simulink model "tta_ut"  (Simulink 8.1)
settings: Solver=ode1  StartTime=0.0  StopTime=Inf  FixedStep=0.001  RelTol=1e-3
PostLoadFcn:
  | , if any(exist('dsrtsu_mdlpostloadfcn', 'file') == [2, 3, 6]), try dsrtsu_mdlpostloadfcn('Execute', bdroot); catch fprintf('Error in PostLoadFcn (dsrtsu_mdlpostloadfcn) for model "%s":\n %s\n', bdroot, lasterr); end, end,
undefined symbols (not defined in the file or in its folder): KIFO_OffsetToBumper_m
libraries: siltestlib x5, tta x1
settings Model: DSRTSU_INTERNAL_RTI_VER=450  DSRTSU_INTERNAL_RTI_TYPE=rti1401  RTICANMMDATA=struct('GeneralSetupData',struct('modelroot','D:\PROJECTS\HAITEC\TAIWAN_HAITEC_SVN\trunk\AdasDragon\software\sw_development\arch\app\ifo','generalsettings',struct('filesettings',struct('destfolder',struct('Name','RTICANMM_FILES','Check',1),'buildfolder',struct('Name','.','Check',1),'AbsDestfolder',struct('Name','D:\PROJECTS\HAITEC\TAIWAN_HAITEC_SVN\trunk\AdasDragon\software\sw_development\arch\app\ifo\RTICANMM_FILES'),'AbsBuildfolder',struct('Name','D:\PROJECTS\HAITEC\TAIWAN_HAITEC_SVN\trunk\AdasDragon\software\sw_development\arch\app\ifo'))),'options',struct('addpaths',1,'rmpaths',1,'addtrcexclusion',logical(1),'cannavigator',struct('checkmonitoring',0),'show_usrtrc',0,'use_usrtrc',0),'advanced',struct('options',[1 1 1 1 1 1 1 1 1 1 1 1 1 1 1 1 1 1 1 1 1 1 1 1 1 1 1 1 1 1 1 1 1 1 1 1 1 1 1 1 1 1 1 1 1 1 1 1 1 1 1 1 1 1 1 1 1 1 1 1 1 1 1 1 1 1 1 1 1 1 1 1 1 1 1 1 1 1 1 1 1 1 1 1 1 1 1 1 1 1 1 1 1 1 1 1 1 1 1 1]),'MPSetup',{{}},'modelname','tta_ut','block','tta_ut'))  DSRTSU_INTERNAL_RTIFPGA=40  Creator=tescamilla  LastModifiedBy=tescamilla  BufferReuse=off
settings DataIOCC: SignalLoggingSaveFormat=Dataset
settings OptimizationCC: BlockReduction=off  OptimizeBlockIOStorage=off  BufferReuse=off  ExpressionFolding=off  ExpressionDepthLimit=128  LocalBlockOutputs=off
settings DebuggingCC: FcnCallInpInsideContextMsg=EnableAllAsError
settings HardwareCC: ProdIntDivRoundTo=Zero  ProdEndianess=BigEndian  ProdHWDeviceType=Generic->Custom  TargetIntDivRoundTo=Zero  TargetEndianess=BigEndian  TargetHWDeviceType=Generic->Custom
settings RTWCC: SystemTargetFile=rti1401.tlc  MakeCommand=make_rti  TemplateMakefile=rti1401.tmf  Description=dSPACE DS1401 Hardware Platform  ProcessScript=rti1401_make_rtw_hook
settings STFCustomTargetCC: CodeReplacementLibrary=ANSI_C  ParMdlRefBuildCompliant=on  GeneratePreprocessorConditionals=Disable all  MatFileLogging=on  SystemTargetFile=rti1401.tlc
settings GRTTargetCC: CompOptLevelCompliant=off  ConcurrentExecutionCompliant=off  ExtModeMexFile=noextcomm
settings CustomProperty: DataType=RTWOptions_EnumType_C__Program Files (x86)_dSPACE RCPHIL 2014-B_MATLAB_RTI_RTI1401_TLC_rti1401_1InitialSimState  Value=RUN
settings EnumStrPairs: String=RUN

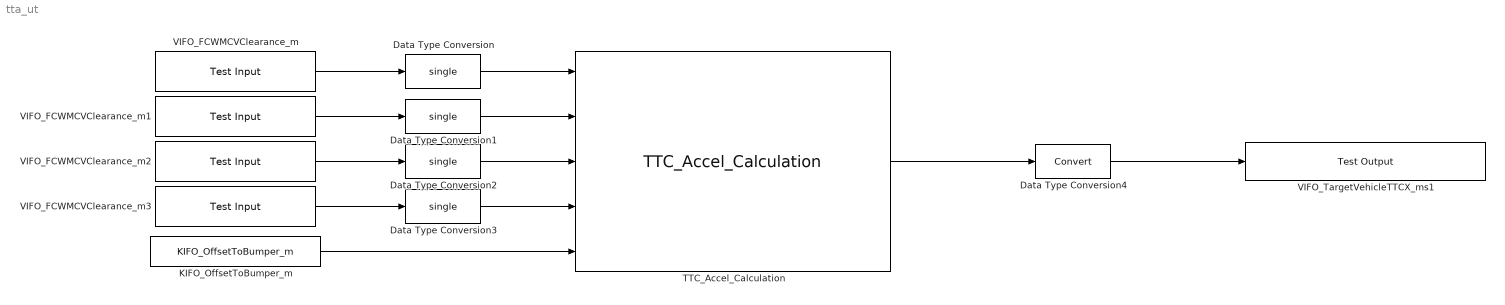
== system tta_ut ==
  Data Type Conversion{,1..3} (4 alike) : DataTypeConversion  OutDataTypeStr=single
  Data Type Conversion4 : DataTypeConversion
  KIFO_OffsetToBumper_m : Constant  Value=KIFO_OffsetToBumper_m
  TTC_Accel_Calculation : tta/TTC_Accel_Calculation
  VIFO_FCWMCVClearance_m : siltestlib/Test Input  varname=Distance_m  sampletime=-1
  VIFO_FCWMCVClearance_m1 : siltestlib/Test Input  varname=RelSpeed_mps  sampletime=-1
  VIFO_FCWMCVClearance_m2 : siltestlib/Test Input  varname=TargetVehAccel_mps2  sampletime=-1
  VIFO_FCWMCVClearance_m3 : siltestlib/Test Input  varname=HostVehAccel_mps2  sampletime=-1
  VIFO_TargetVehicleTTCX_ms1 : siltestlib/Test Output  varname=EnhancedTtc_ms  sampletime=-1
  wires:
  VIFO_FCWMCVClearance_m/1 -> Data Type Conversion/1
  Data Type Conversion/1 -> TTC_Accel_Calculation/1
  VIFO_FCWMCVClearance_m1/1 -> Data Type Conversion1/1
  Data Type Conversion1/1 -> TTC_Accel_Calculation/2
  VIFO_FCWMCVClearance_m2/1 -> Data Type Conversion2/1
  Data Type Conversion2/1 -> TTC_Accel_Calculation/3
  VIFO_FCWMCVClearance_m3/1 -> Data Type Conversion3/1
  Data Type Conversion3/1 -> TTC_Accel_Calculation/4
  TTC_Accel_Calculation/1 -> Data Type Conversion4/1
  Data Type Conversion4/1 -> VIFO_TargetVehicleTTCX_ms1/1
  KIFO_OffsetToBumper_m/1 -> TTC_Accel_Calculation/5
